simulink model "SimpleSystemSimulation"  (R2022b)
settings: Solver=VariableStepAuto  StartTime=0.0  StopTime=50.0  MaxStep=0.1  RelTol=1e-3
settings Model: Creator=lang lang  LastModifiedBy=lang lang

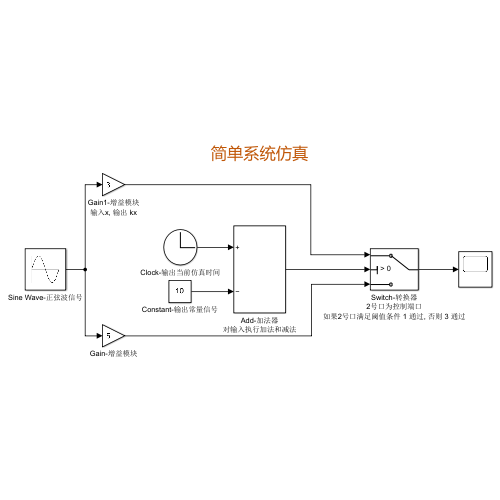
[thumbnail: Simulink's stored preview of the top-level diagram]
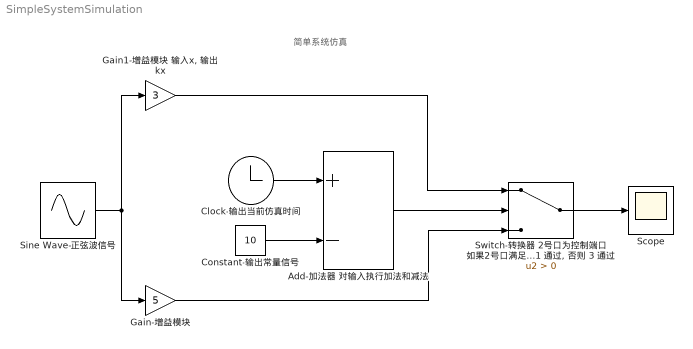
== system SimpleSystemSimulation ==
  note: 简单系统仿真
  Add-加法器 对输入执行加法和减法 : Sum  Inputs=+-
  Clock-输出当前仿真时间 : Clock
  Constant-输出常量信号 : Constant  Value=10
  Gain-增益模块 : Gain  Gain=5
  "Gain1-增益模块 输入x, 输出 kx" : Gain  Gain=3
  Scope : Scope
  Sine Wave-正弦波信号 : Sin  SampleTime=0
  "Switch-转换器 2号口为控制端口 如果2号口满足阈值条件 1 通过, 否则 3 通过" : Switch  Criteria=u2 > Threshold  SaturateOnIntegerOverflow=off  InputSameDT=off
  wires:
  Clock-输出当前仿真时间/1 -> Add-加法器 对输入执行加法和减法/1
  Sine Wave-正弦波信号/1 -> "Gain1-增益模块 输入x, 输出 kx"/1, Gain-增益模块/1
  Constant-输出常量信号/1 -> Add-加法器 对输入执行加法和减法/2
  Add-加法器 对输入执行加法和减法/1 -> "Switch-转换器 2号口为控制端口 如果2号口满足阈值条件 1 通过, 否则 3 通过"/2
  "Gain1-增益模块 输入x, 输出 kx"/1 -> "Switch-转换器 2号口为控制端口 如果2号口满足阈值条件 1 通过, 否则 3 通过"/1
  Gain-增益模块/1 -> "Switch-转换器 2号口为控制端口 如果2号口满足阈值条件 1 通过, 否则 3 通过"/3
  "Switch-转换器 2号口为控制端口 如果2号口满足阈值条件 1 通过, 否则 3 通过"/1 -> Scope/1
